simulink model "EarlyReturn13"  (R2020b)
settings: Solver=VariableStepAuto  StartTime=0.0  StopTime=0.1  RelTol=1e-3
settings Model: Creator=BEAR  LastModifiedBy=apple
settings DataIOCC: ReturnWorkspaceOutputs=off
settings DebuggingCC: ArithmeticOperatorsInVariantConditions=warning
settings SFSimCC: SimUseLocalCustomCode=off  CustomCodeUndefinedFunction=UseInterfaceOnly
settings RTWCC: RTWUseLocalCustomCode=off

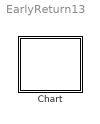
== system EarlyReturn13 ==
  Chart : Stateflow chart  TreatAsAtomicUnit=on

== stateflow chart EarlyReturn13/Chart ==
  state A [parallel]
    settings: executionOrder=1
    state A1
      ex: fprintf("exA1");
      x=x-1;E;
      fprintf("exA1_done")
    state A2
      en: fprintf("enA2")
    state A3
      en: fprintf("enA3")
    (default) -> A1 : {x=5;}
    A1 -> A2 [order 2] : F
    A1 -> A3 [order 1] : E[x>0]
  state B [parallel]
    settings: executionOrder=2
    state B1
    state B2
    (default) -> B1
    B1 -> B2 : /{fprintf("F");F}
  data: x local
  events: E local FUNCTION_CALL_EVENT; F local FUNCTION_CALL_EVENT
